simulink model "HandsON_2"  (R2023b)
settings: Solver=FixedStepAuto  StartTime=0.0  StopTime=t_end  FixedStep=1  RelTol=1e-3
undefined symbols (not defined in the file): alpha_1, alpha_2, beta_3, delta_1, delta_2, gamma_3
settings Model: Creator=alberto  LastModifiedBy=alberto

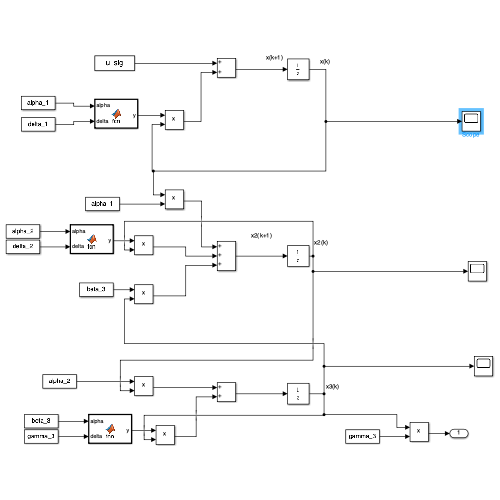
[thumbnail: Simulink's stored preview of the top-level diagram]
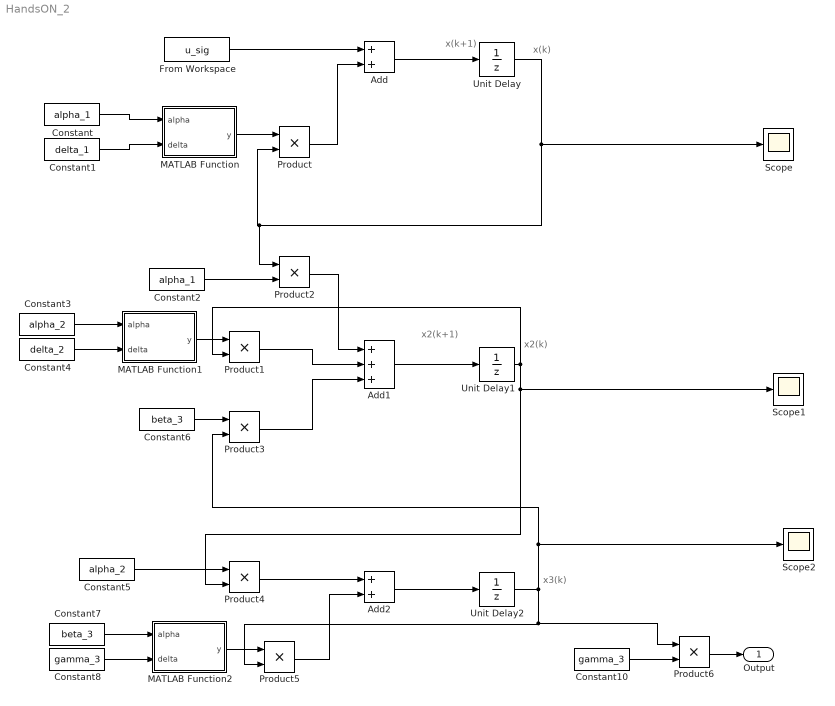
== system HandsON_2 ==
  note: x3(k)
  note: x2(k)
  note: x2(k+1)
  note: x(k)
  note: x(k+1)
  Add : Sum
  Add1 : Sum  Inputs=+++
  Add2 : Sum
  Constant : Constant  Value=alpha_1
  Constant1 : Constant  Value=delta_1
  Constant10 : Constant  Value=gamma_3
  Constant2 : Constant  Value=alpha_1
  Constant3 : Constant  Value=alpha_2
  Constant4 : Constant  Value=delta_2
  Constant5 : Constant  Value=alpha_2
  Constant6 : Constant  Value=beta_3
  Constant7 : Constant  Value=beta_3
  Constant8 : Constant  Value=gamma_3
  From Workspace : FromWorkspace  VariableName=u_sig
  MATLAB Function : MATLAB Function  TreatAsAtomicUnit=on
  MATLAB Function1 : MATLAB Function  TreatAsAtomicUnit=on
  MATLAB Function2 : MATLAB Function  TreatAsAtomicUnit=on
  Product{,1..6} (7 alike) : Product
  Scope : Scope
  Scope1 : Scope
  Scope2 : Scope
  Unit Delay : UnitDelay  SampleTime=-1  HasFrameUpgradeWarning=on
  Unit Delay1 : UnitDelay  SampleTime=-1  HasFrameUpgradeWarning=on
  Unit Delay2 : UnitDelay  SampleTime=-1  HasFrameUpgradeWarning=on
  Output : Outport
  wires:
  From Workspace/1 -> Add/1
  Constant/1 -> MATLAB Function/1(alpha)
  Constant1/1 -> MATLAB Function/2(delta)
  MATLAB Function/1(y) -> Product/1
  Unit Delay/1 -> Product2/1, Product/2, Scope/1
  Add/1 -> Unit Delay/1
  Product/1 -> Add/2
  MATLAB Function1/1(y) -> Product1/1
  Product1/1 -> Add1/2
  Add1/1 -> Unit Delay1/1
  Unit Delay1/1 -> Product4/2, Scope1/1, Product1/2
  Constant2/1 -> Product2/2
  Product2/1 -> Add1/1
  Constant6/1 -> Product3/1
  Unit Delay2/1 -> Scope2/1, Product3/2, Product6/1, Product5/2
  Product3/1 -> Add1/3
  Constant3/1 -> MATLAB Function1/1(alpha)
  Constant4/1 -> MATLAB Function1/2(delta)
  Add2/1 -> Unit Delay2/1
  Constant5/1 -> Product4/1
  Product4/1 -> Add2/1
  Constant7/1 -> MATLAB Function2/1(alpha)
  Constant8/1 -> MATLAB Function2/2(delta)
  MATLAB Function2/1(y) -> Product5/1
  Product5/1 -> Add2/2
  Constant10/1 -> Product6/2
  Product6/1 -> Output/1

== matlab function HandsON_2/MATLAB Function ==
  data: alpha input; y output; delta input
function y = fcn(alpha, delta)

y = 1 - alpha - delta;

== matlab function HandsON_2/MATLAB Function2 ==
  data: alpha input; y output; delta input
function y = fcn(alpha, delta)

y = 1 - alpha - delta;

== matlab function HandsON_2/MATLAB Function1 ==
  data: alpha input; y output; delta input
function y = fcn(alpha, delta)

y = 1 - alpha - delta;
